simulink model "IslandMode"  (R2022b)
settings: Solver=ode23tb  StartTime=0.0  StopTime=24*3600*365*3  FixedStep=60  RelTol=1e-3
values from neighbouring files (symbols this model uses):
  Fnom = 50    [run_test.m]
  OverChargingProtection = 0    [run_test.m]
  Tsample = 60    [run_test.m]
  Vnom = sqrt(3)*230    [run_test.m]
libraries: simulink x12, ET3036TU_model_library_2021b x7, spsThreePhaseDynamicLoadLib x3, spspowerguiLib x1
settings Model: Creator=nkpanda  LastModifiedBy=jeroen
settings SolverCC: ZeroCrossAlgorithm=Adaptive
settings DebuggingCC: IgnoredZcDiagnostic=none  UnconnectedInputMsg=warning  UnconnectedOutputMsg=warning  UnconnectedLineMsg=warning
settings ModelReferenceCC: EnableRefExpFcnMdlSchedulingChecks=on
settings RTWCC: DLArmComputeVersion=19.05

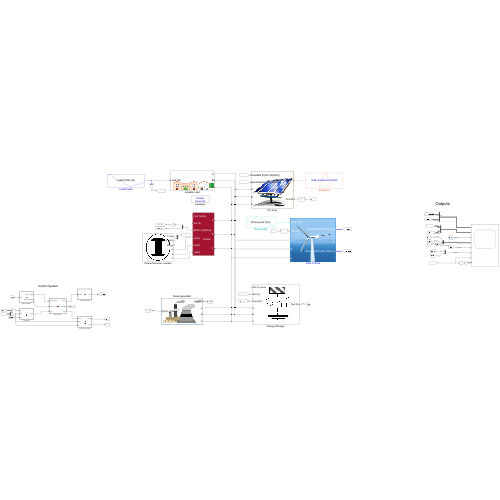
[thumbnail: Simulink's stored preview of the top-level diagram]
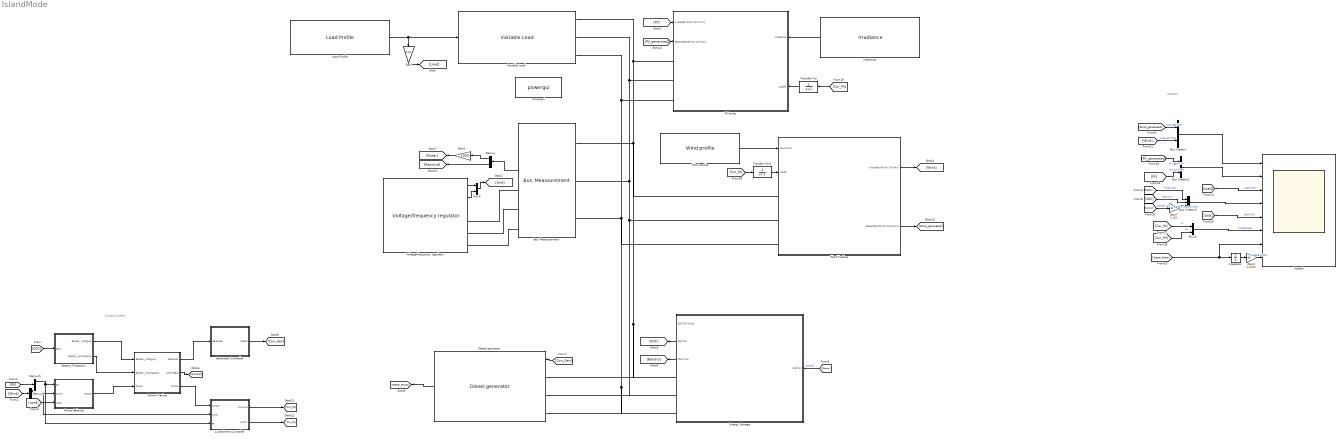
== system IslandMode ==
  note: Control System
  note: Outputs
  Battery Protection : MATLAB Function  TreatAsAtomicUnit=on
  Bus Creator : BusCreator  Inputs=2
  Bus Creator1 : BusCreator  Inputs=2
  Bus Creator2 : BusCreator  Inputs=3
  "Bus Meassurement " : ET3036TU_model_library_2021b/Bus  Meassurement 
  Curtailment Controller : MATLAB Function  TreatAsAtomicUnit=on
  Demux : Demux  Outputs=2
  Demux5 : Demux  Outputs=2
  Demux6 : Demux  Outputs=2
  Diesel generator : ET3036TU_model_library_2021b/Diesel generator  Snom=150  Pfactor=1
  Energy Storage : Subsystem  AncestorBlock=ET3036TU_model_library_2021b/Energy Storage  mask(Grid-connected Energy Storage (PQ Model)){Vn=Vnom, Fn=Fnom, PnomkW=150, kWh_Rated=651.78, Efficiency=100, LimitVec=[90 10], RechargeSOC=70, Precharge=100, autoRecharge=off, Initial_kWh_pc=50, PQvec=[0 0], ovrchargpro=OverChargingProtection}
      mask prompts: Vn "Nominal Line Voltage [Vrms]"; Fn "Nominal Frequency [Hz]"; PnomkW "Rated Power [kW]"; kWh_Rated "Rated Capacity [kWh]"; Efficiency "Overall System Efficiency [%]"; LimitVec "Upper/Lower Charge Limits [%]"; RechargeSOC "SOC to Recharge [%]"; Precharge "Recharge Rate [% of Rated Power]"; autoRecharge "Enable Auto-Recharge"; Initial_kWh_pc "Initial State-of-Charge [0-100%]"; PQvec "Initial Active/Reactive Cmds"; ovrchargpro "Enable over charging/ discharging protection (0: Disable, 1: Enable)"
      mask help:
      | The energy storage block models a generic grid-connected energy storage system (ESS), most commonly a battery system. This is a system-level model that does not contain any power electronics, but is useful for load flow, phasor, and hybrid phasor-EMT simulations. The inputs to this block are the commanded active and reactive power of the ESS.
      |
      | Note: Positive cmd indicates discharging (supply), negative cmd indicates charging (load).
      | Note: The initial active/reactive power commands must be specified for use for Load Flow analysis.
      mask init:
      | % Calculate Initial Conditions
      | Pnom = PnomkW*1e3;
      | P0 = -PQvec(1);  Q0 = -PQvec(2);
      | if abs(P0) > Pnom
      |     P0 = sign(P0)*Pnom;
      | end
      | 
      | % Calculate Q0 given Reactive Power Capability Curve
      | Qlim = sqrt(Pnom^2 - P0^2);
      | if Qlim > abs(Q0)
      |     Q0 = sign(Q0)*Qlim;
      | end
      | 
      | UpChrgLim = LimitVec(1);
      | LowChrgLim = LimitVec(2);
      | if Initial_kWh_pc > UpChrgLim && P0 < 0
      |     P0 = 0; Q0 = 0;
      | elseif Initial_kWh_pc < LowChrgLim && P0 > 0
      |     P0 = 0; Q0 = 0;
      | end
      settings: LibrarySourceBlock=ET3036TU_model_library_2021b/Energy Storage
      mask DialogControl Container7 Prompt: Grid Connection Properties
      mask DialogControl Container11 Prompt: Charge/Discharge Controls
      mask DialogControl Container12 Prompt: Initial Conditions
      mask Display: image('$imagefile'); % Use "Edit Image" on toolstrip to change.
  Gain : Gain  Gain=0.001
  Gain1 : Gain  Gain=1000
  Gain2 : Gain  Gain=1/3600
  Gain7 : Gain  Gain=0.001
  Generator Controller : MATLAB Function  TreatAsAtomicUnit=on
  Integrator : Integrator
  Irradiance : ET3036TU_model_library_2021b/Irradiance
  Load Profile : ET3036TU_model_library_2021b/Load Profile
  Mux4 : Mux  Inputs=2
  Mux5 : Mux  Inputs=2
  "PV array " : Subsystem  AncestorBlock=ET3036TU_model_library_2021b/PV array  mask(PV farm){Efficiency=0.2, Area=822.71, Vnom=Vnom, fnom=Fnom}
      mask prompts: Efficiency "Total efficiency (fraction)"; Area "Area (m2)"; Vnom "Rated Line voltage (Vrms)"; fnom "Rated frequency (Hz):"
      mask help: The product of the efficiency, the area covered by the PV farm and the irradiance in W/m2 will give you the power generated by the PV farm.
      settings: LibrarySourceBlock=ET3036TU_model_library_2021b/PV array
      mask Display:
      | color('white')
      | image(imread('pv.jpg'))
      | 
      | color('black')
      | port_label('RConn',1,'A')
      | port_label('RConn',2,'B')
      | port_label('RConn',3,'C')
      | port_label('output',1,'Available [P(kW) Q(kVAr)]')
      | port_label('output',2,'Generated [P(kW) Q(kVAr)]')
      | 
      | port_label('input',1,'Irradiance (W/m2)')
      | port_label('input',2,'Cut-off')
  Power Balance : MATLAB Function  TreatAsAtomicUnit=on
  Power Tracker : MATLAB Function  TreatAsAtomicUnit=on
  Scope3 : Scope  NumInputPorts=8
  Transfer Fcn : TransferFcn  Denominator=[1 1]
  Transfer Fcn1 : TransferFcn  Denominator=[1 1]
  Variable Load : ET3036TU_model_library_2021b/Variable Load  PF=1  Load0=0
  Voltage/frequency regulator : ET3036TU_model_library_2021b/Voltage//frequency regulator
  "Wind Turbine " : Subsystem  AncestorBlock=ET3036TU_model_library_2021b/Wind Turbine  mask{Unom=15, Umax=25, Umin=3, Pselect=1: Simple Cubic Power, fnom=Fnom, Vnom=Vnom, Pnom=226.56, rp=5, Cp=16/27, rho=1.225, Uvec=1:1:30, Pvec=[0,0,0,0,21359.3750000000,58193.5000000000,104316.125000000,157104.500000000,213935.875000000,272187.500000000,329236.625000000,382460.500000000,429236.375000000,466941.500000000,492953.125000000,500000,500000,500000,500000,500000,500000,500000,500000,500000,500000,0,0,0,0,0], Tp=1, Tq=0.1, ReactP=0}
      mask prompts: Unom "Nominal Wind Speed [m/s]"; Umax "Maximum Operating Wind [m/s]"; Umin "Minimum Operating Wind [m/s]"; Pselect "Wind Turbine Power Model"; fnom "Nominal frequency (Hz):"; Vnom "Nominal phae-to-phase voltage (Vrms)"; Pnom "Nominal Power, [kW]"; rp "Blade Radius, r [m]"; Cp "Performance Coefficient, Cp"; rho "Air Density, rho [kg/m^3]"; Uvec "Wind Vec [m/s]"; Pvec "Power Vec [W]"; Tp "Active Power Dynamics, Tp [s]"; Tq "Reactive Power Dynamics, Tq [s]"; ReactP "Reactive Power Percentage [%]"
      mask help:
      | Simple Wind Turbine that serves as an Active and Reactive Power Source depending on the Wind Power Curve.
      |
      | The Wind Turbine Power Curve can be defined by one of three models:
      | 1: Simple cubic power curve
      | 2: Physical wind turbine parameters
      | 3: Look-up table (from a wind turbine data sheet).
      |
      | Cutoff takes value 1 or 0. 1 denotes manual forced cut-off od wind power generation even though potnetial wind power is available
      | The 'General' and 'Dynamics' tabs apply to all models.
      mask init:
      | A = pi*rp^2;
      | 
      | if Pselect == 1,
      |     Pmax = Pnom*1e3;
      | elseif Pselect == 2,
      |     Pmax = 1/2*rho*Cp*A*Umax^3;
      | else
      |     Pmax = max(Pvec);
      | end
      | Qmax = (ReactP/100)*Pmax;
      settings: LibrarySourceBlock=ET3036TU_model_library_2021b/Wind Turbine
      mask TypeOptions Pselect: 1: Simple Cubic Power | 2: Physical parameters | 3: Look-up Fit
      mask DialogControl Container4 Prompt: General
      mask DialogControl Container16 Prompt: Turbine
      mask DialogControl Container10 Prompt: Electrical
      mask DialogControl Container12 Prompt: 1: Cubic
      mask DialogControl Container9 Prompt: 2: Physical
      mask DialogControl Container7 Prompt: 3: Lookup
      mask DialogControl Container8 Prompt: Dynamics
      mask Display:
      | image(imread('eolienne.bmp'))
      | 
      | color('white')
      | port_label('LConn',1,'A')
      | port_label('LConn',2,'B')
      | port_label('LConn',3,'C')
      | 
      | port_label('output',1,'Available [P(kW) Q(kVAr)]')
      | port_label('output',2,'Generated [P(kW) Q(kVAr)]')
      | port_label('input',1,'Wind (m/s)')
      | port_label('input',2,'Cut-off')
  Wind profile : ET3036TU_model_library_2021b/Wind profile
  powergui : spspowerguiLib/powergui  Priority=1  SimulationMode=Phasor  SampleTime=Tsample  frequency=Fnom  Iterations=50  frequencyindice=50  Pbase=100e6  ErrMax=1e-4  UnitsV=kV  UnitsW=MW  buscounter=0  FunctionMessages=off  echomessages=off  EnableUseOfTLC=off  CurrentSourceSwitches=off  DisableSnubberDevices=off  DisableRonSwitches=off  DisableVfSwitches=off  DisplayEquations=off  AutomaticDiscreteSolvers=off  SolverType=Tustin/Backward Euler (TBE)  Interpol=off  ExternalGateDelay=off  methode=off  Ts=100  x0status=blocks  SPID=on  SwTol=0  HookPort=off  NonlinearTolerance=1e-4  nMaxIteration=100  ContinueOnMaxIteration=off  RestoreLinks=warning  ResistiveCurrentMeasurement=off  Frange=[0:2:500]  Ylog=off  Xlog=on  ShowGrid=off  save=off  variable=ZData  structure=0  ZoomFFT=off  StartTime=0.0  cycles=1  DisplayStyle=1  fundamental=60  FreqAxis=off  MaxFrequency=1000  frequencyindicesteady=1  RmsSteady=1  display=off
  wires:
  Load Profile/1 -> Gain/1, Variable Load/1
  Irradiance/1 -> "PV array "/1(Irradiance)
  Energy Storage/3(Pout (kW)) -> [Battery]
  Energy Storage/2(SOC(%)) -> [SOC]
  Gain/1 -> [Load]
  [Control] -> Energy Storage/1(Pref (W))  "Control"
  Demux/1 -> Gain1/1
  Gain1/1 -> [Power]
  "Bus Meassurement "/3 -> Demux/1
  Demux/2 -> [Reactive]
  [Cur_PV] -> Transfer Fcn/1
  [Cur_W] -> Transfer Fcn1/1
  "PV array "/1(Available [P(kW) Q(kVAr)]) -> [PV]
  "Wind Turbine "/1(Available [P(kW) Q(kVAr)]) -> [Wind]
  Transfer Fcn/1 -> "PV array "/2(cutoff1)
  Transfer Fcn1/1 -> "Wind Turbine "/2(cutoff)
  [Battery] -> Bus Creator2/1  "P_bat (kW)"
  [SOC] -> Bus Creator2/2  "SOC (%)"
  "Wind Turbine "/2(Generated [P(kW) Q(kVAr)]1) -> [Wind_generated]
  "PV array "/2(Generated [P(kW) Q(kVAr)]) -> [PV_generated]
  [Wind_generated] -> Bus Creator/1  "wind_gen(kW)"
  [Wind] -> Bus Creator/2  "wind_act (kW)"
  [PV] -> Bus Creator1/2  "PV_act (kW)"
  [PV_generated] -> Bus Creator1/1  "PV_gen (kW)"
  Bus Creator/1 -> Scope3/1
  Bus Creator1/1 -> Scope3/2
  Bus Creator2/1 -> Scope3/4
  [Control] -> Gain7/1  "Control (W)"
  Gain7/1 -> Bus Creator2/3  "Battery Control (kW)"
  [Cur_W] -> Mux4/1  "W"
  [Cur_PV] -> Mux4/2  "PV"
  Mux4/1 -> Scope3/6  "Curtailment"
  [SOC] -> Battery Protection/1(SOC)
  [Load] -> Power Balance/3(Load)
  Battery Protection/1(Battery_charging) -> Power Tracker/1(Battery_Charging)
  Power Balance/1(Power) -> Power Tracker/3(Power)
  Power Tracker/3(Curtail) -> Curtailment Controller/1(Curtail)
  Power Tracker/1(Generate) -> Generator Controller/1(Generate)
  Curtailment Controller/1(Curwind) -> [Cur_W]
  Curtailment Controller/2(CurPV) -> [Cur_PV]
  [PV] -> Demux5/1
  Demux5/1 -> Curtailment Controller/3(PV), Power Balance/1(Sol)
  [Wind] -> Demux6/1
  Demux6/1 -> Curtailment Controller/2(wind), Power Balance/2(Wind)
  Battery Protection/2(Battery_discharging) -> Power Tracker/2(Battery_discharging)
  [Load] -> Scope3/3  "Load (kW)"
  [Grid] -> Scope3/5  "Grid (kW)"
  Generator Controller/1(Diesel) -> [Con_Gen]
  Diesel generator/1 -> [Diesel_Power]
  [Diesel_Power] -> Scope3/7, Integrator/1
  Wind profile/1 -> "Wind Turbine "/1(Wind (m/s))
  [Con_Gen] -> Diesel generator/1
  Voltage/frequency regulator/1 -> Mux5/1
  Voltage/frequency regulator/2 -> Mux5/2
  Mux5/1 -> [Grid]
  Integrator/1 -> Gain2/1
  Gain2/1 -> Scope3/8  "Diesel (kWh)"
  Power Tracker/2(ControlBat) -> [Control]
  connections:
  "Bus Meassurement "/RConn1 -- Voltage/frequency regulator/RConn1
  "Bus Meassurement "/RConn2 -- Voltage/frequency regulator/RConn2
  "Bus Meassurement "/RConn3 -- Voltage/frequency regulator/RConn3
  "PV array "/RConn2 -- Energy Storage/RConn2 -- Diesel generator/LConn2 -- "Wind Turbine "/LConn2 -- "Bus Meassurement "/LConn2 -- Variable Load/RConn2
  "Bus Meassurement "/LConn1 -- "Wind Turbine "/LConn1 -- Diesel generator/LConn1 -- Energy Storage/RConn1 -- Variable Load/RConn1 -- "PV array "/RConn1
  "PV array "/RConn3 -- "Wind Turbine "/LConn3 -- Diesel generator/LConn3 -- Energy Storage/RConn3 -- "Bus Meassurement "/LConn3 -- Variable Load/RConn3

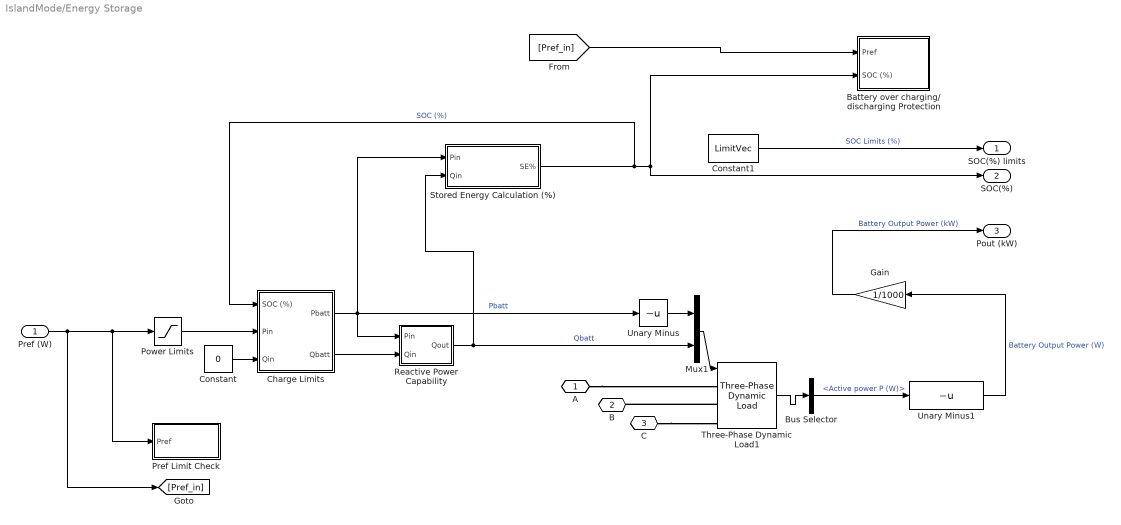
== system IslandMode/Energy Storage ==
  Pref (W) : Inport
  Battery over charging/ discharging Protection : Subsystem
  Bus Selector : BusSelector  OutputSignals=Active power P (W)
  Charge Limits : Subsystem
  Constant : Constant  Value=0
  Constant1 : Constant  Value=LimitVec
  Gain : Gain  Gain=1/1000
  Mux1 : Mux  Inputs=2
  Power Limits : Saturate  UpperLimit=Pnom  LowerLimit=-Pnom
  Pref Limit Check : Subsystem
  Reactive Power Capability : Subsystem
  Stored Energy Calculation (%) : Subsystem
  Three-Phase Dynamic Load1 : spsThreePhaseDynamicLoadLib/Three-Phase Dynamic Load  NominalVoltage=[Vn Fn]  ActiveReactivePowers="[ 0  0]"  PositiveSequence=[Vn 0]  ExternalControl=on  NpNq=[1.3 2]  TimeConstants="[0  0  0  0]"  MinimumVoltage=0.7  Tfilter=1e-4  LoadFlowParameters=[4,0,0,0,0]
  Unary Minus : UnaryMinus
  Unary Minus1 : UnaryMinus
  A : PMIOPort  Side=Right
  B : PMIOPort  Port=2  Side=Right
  C : PMIOPort  Port=3  Side=Right
  SOC(%) limits : Outport  VectorParamsAs1DForOutWhenUnconnected=off
  SOC(%) : Outport  Port=2  VectorParamsAs1DForOutWhenUnconnected=off
  Pout (kW) : Outport  Port=3  VectorParamsAs1DForOutWhenUnconnected=off
  wires:
  Unary Minus/1 -> Mux1/1
  Mux1/1 -> Three-Phase Dynamic Load1/1
  Three-Phase Dynamic Load1/1 -> Bus Selector/1
  Reactive Power Capability/1(Qout) -> Stored Energy Calculation (%)/2(Qin), Mux1/2  "Qbatt"
  Pref (W)/1 -> [Pref_in], Pref Limit Check/1(Pref), Power Limits/1
  Stored Energy Calculation (%)/1(SE%) -> Battery over charging/ discharging Protection/2(SOC (%)), SOC(%)/1, Charge Limits/1(SOC (%))  "SOC (%)"
  Charge Limits/1(Pbatt) -> Stored Energy Calculation (%)/1(Pin), Unary Minus/1, Reactive Power Capability/1(Pin)  "Pbatt"
  Power Limits/1 -> Charge Limits/2(Pin)
  Constant/1 -> Charge Limits/3(Qin)
  Charge Limits/2(Qbatt) -> Reactive Power Capability/2(Qin)
  Bus Selector/1 -> Unary Minus1/1  "<Active power P (W)>"
  Unary Minus1/1 -> Gain/1  "Battery Output Power (W)"
  Gain/1 -> Pout (kW)/1  "Battery Output Power (kW)"
  [Pref_in] -> Battery over charging/ discharging Protection/1(Pref)
  Constant1/1 -> SOC(%) limits/1  "SOC Limits (%)"
  connections:
  Three-Phase Dynamic Load1/LConn2 -- B/RConn1
  C/RConn1 -- Three-Phase Dynamic Load1/LConn3
  A/RConn1 -- Three-Phase Dynamic Load1/LConn1

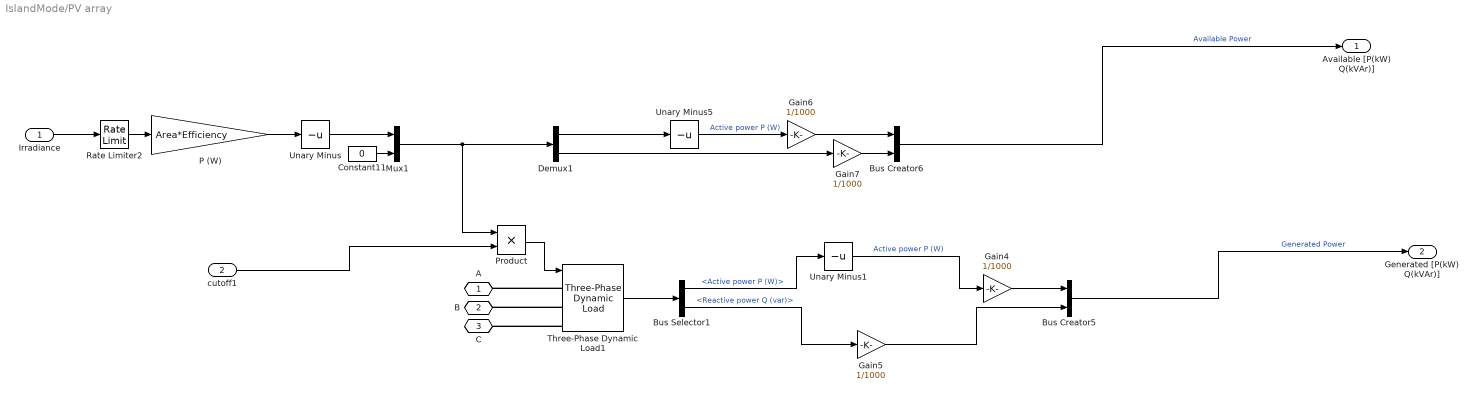
== system IslandMode/PV array  ==
  Irradiance : Inport
  cutoff1 : Inport  Port=2
  Bus Creator5 : BusCreator  Inputs=2
  Bus Creator6 : BusCreator  Inputs=2
  Bus Selector1 : BusSelector  OutputSignals=Active power P (W),Reactive power Q (var)
  Constant11 : Constant  Value=0
  Demux1 : Demux  Outputs=2
  Gain{4..7} (4 alike) : Gain  Gain=1/1000
  Mux1 : Mux  Inputs=2
  P (W) : Gain  Gain=Area*Efficiency
  Product : Product
  Rate Limiter2 : RateLimiter  RisingSlewLimit=1e4  FallingSlewLimit=-1e4  SampleTimeMode=inherited
  Three-Phase Dynamic Load1 : spsThreePhaseDynamicLoadLib/Three-Phase Dynamic Load  NominalVoltage=[Vnom fnom]  ActiveReactivePowers="[ 0  0]"  PositiveSequence=[Vnom 0]  ExternalControl=on  NpNq=[1.3 2]  TimeConstants="[0  0  0  0]"  MinimumVoltage=0.7  Tfilter=1e-4  LoadFlowParameters=[4,0,0,0,0]
  Unary Minus : UnaryMinus
  Unary Minus1 : UnaryMinus
  Unary Minus5 : UnaryMinus
  A : PMIOPort  Side=Right
  B : PMIOPort  Port=2  Side=Right
  C : PMIOPort  Port=3  Side=Right
  Available [P(kW) Q(kVAr)] : Outport  VectorParamsAs1DForOutWhenUnconnected=off
  Generated [P(kW) Q(kVAr)] : Outport  Port=2  VectorParamsAs1DForOutWhenUnconnected=off
  wires:
  Bus Creator5/1 -> Generated [P(kW) Q(kVAr)]/1  "Generated Power"
  Rate Limiter2/1 -> P (W)/1
  Constant11/1 -> Mux1/2
  Unary Minus/1 -> Mux1/1
  P (W)/1 -> Unary Minus/1
  Irradiance/1 -> Rate Limiter2/1
  Bus Selector1/1 -> Unary Minus1/1  "<Active power P (W)>"
  Unary Minus1/1 -> Gain4/1  "Active power P (W)"
  Three-Phase Dynamic Load1/1 -> Bus Selector1/1
  Bus Selector1/2 -> Gain5/1  "<Reactive power Q (var)>"
  Gain4/1 -> Bus Creator5/1
  Gain5/1 -> Bus Creator5/2
  Demux1/1 -> Unary Minus5/1
  Gain6/1 -> Bus Creator6/1
  Demux1/2 -> Gain7/1
  Unary Minus5/1 -> Gain6/1  "Active power P (W)"
  Gain7/1 -> Bus Creator6/2
  Bus Creator6/1 -> Available [P(kW) Q(kVAr)]/1  "Available Power"
  Product/1 -> Three-Phase Dynamic Load1/1
  Mux1/1 -> Product/1, Demux1/1
  cutoff1/1 -> Product/2
  connections:
  Three-Phase Dynamic Load1/LConn2 -- B/RConn1
  Three-Phase Dynamic Load1/LConn1 -- A/RConn1
  Three-Phase Dynamic Load1/LConn3 -- C/RConn1

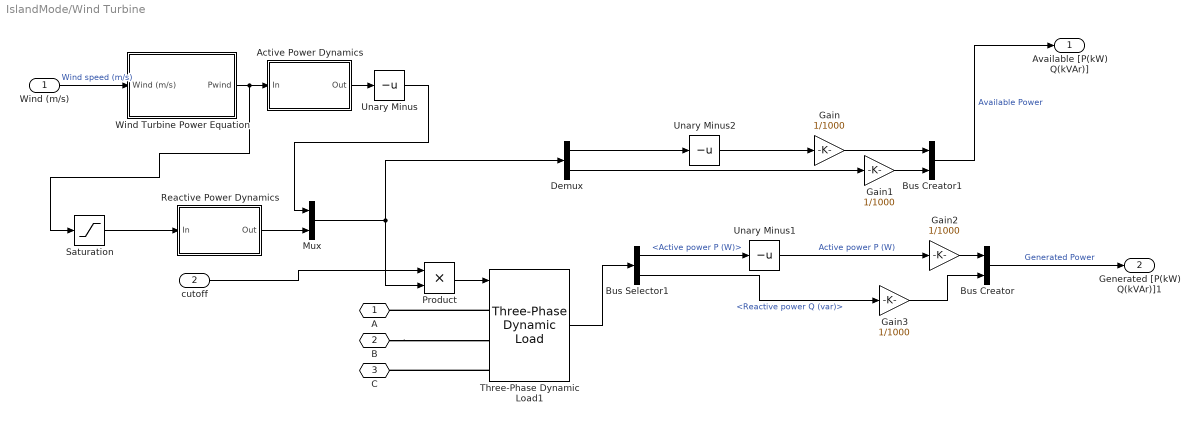
== system IslandMode/Wind Turbine  ==
  Wind (m/s) : Inport
  cutoff : Inport  Port=2
  Active Power Dynamics : Subsystem  VariantControl=T6NotZero
      mask Display: disp('1 / (1 + s T_P)','texmode','on');
  Bus Creator : BusCreator  Inputs=2
  Bus Creator1 : BusCreator  Inputs=2
  Bus Selector1 : BusSelector  OutputSignals=Active power P (W),Reactive power Q (var)
  Demux : Demux  Outputs=2
  Gain{,1..3} (4 alike) : Gain  Gain=1/1000
  Mux : Mux  Inputs=2
  Product : Product
  Reactive Power Dynamics : Subsystem  VariantControl=T6NotZero
      mask Display: disp('1 / (1 + s T_Q)','texmode','on');
  Saturation : Saturate  UpperLimit=Qmax  LowerLimit=-Qmax
  Three-Phase Dynamic Load1 : spsThreePhaseDynamicLoadLib/Three-Phase Dynamic Load  NominalVoltage=[Vnom fnom]  ActiveReactivePowers="[ 0  0]"  PositiveSequence=[Vnom 0]  ExternalControl=on  NpNq=[1.3 2]  TimeConstants="[0  0  0  0]"  MinimumVoltage=0.7  Tfilter=1e-4  LoadFlowParameters=[4,0,0,0,0]
  Unary Minus : UnaryMinus
  Unary Minus1 : UnaryMinus
  Unary Minus2 : UnaryMinus
  Wind Turbine Power Equation : Subsystem
  A : PMIOPort  Side=Left
  B : PMIOPort  Port=2  Side=Left
  C : PMIOPort  Port=3  Side=Left
  Available [P(kW) Q(kVAr)] : Outport  VectorParamsAs1DForOutWhenUnconnected=off
  Generated [P(kW) Q(kVAr)]1 : Outport  Port=2  VectorParamsAs1DForOutWhenUnconnected=off
  wires:
  Bus Selector1/2 -> Gain3/1  "<Reactive power Q (var)>"
  Unary Minus1/1 -> Gain2/1  "Active power P (W)"
  Bus Selector1/1 -> Unary Minus1/1  "<Active power P (W)>"
  Three-Phase Dynamic Load1/1 -> Bus Selector1/1
  Unary Minus/1 -> Mux/1
  Active Power Dynamics/1(Out) -> Unary Minus/1
  Wind Turbine Power Equation/1(Pwind) -> Saturation/1, Active Power Dynamics/1(In)
  Reactive Power Dynamics/1(Out) -> Mux/2
  Saturation/1 -> Reactive Power Dynamics/1(In)
  Wind (m/s)/1 -> Wind Turbine Power Equation/1(Wind (m/s))  "Wind speed (m/s)"
  Mux/1 -> Demux/1, Product/2
  Product/1 -> Three-Phase Dynamic Load1/1
  cutoff/1 -> Product/1
  Demux/1 -> Unary Minus2/1
  Demux/2 -> Gain1/1
  Unary Minus2/1 -> Gain/1
  Gain/1 -> Bus Creator1/1
  Gain1/1 -> Bus Creator1/2
  Gain2/1 -> Bus Creator/1
  Gain3/1 -> Bus Creator/2
  Bus Creator1/1 -> Available [P(kW) Q(kVAr)]/1  "Available Power"
  Bus Creator/1 -> Generated [P(kW) Q(kVAr)]1/1  "Generated Power"
  connections:
  B/RConn1 -- Three-Phase Dynamic Load1/LConn2
  Three-Phase Dynamic Load1/LConn3 -- C/RConn1
  Three-Phase Dynamic Load1/LConn1 -- A/RConn1

== system IslandMode/Energy Storage/Battery over charging// discharging Protection ==
  Pref : Inport
  SOC (%) : Inport  Port=2
  Over Charging Protection : Subsystem
  Under Charging Protection : Subsystem
  wires:
  SOC (%)/1 -> Under Charging Protection/1(SOC (%)), Over Charging Protection/1(SOC (%))
  Pref/1 -> Under Charging Protection/2(Pref), Over Charging Protection/2(Pref)

== system IslandMode/Energy Storage/Charge Limits ==
  SOC (%) : Inport
  Pin : Inport  Port=2
  Qin : Inport  Port=3
  Overcharge Check : Subsystem
  Undercharge Check : Subsystem
  Pbatt : Outport  VectorParamsAs1DForOutWhenUnconnected=off
  Qbatt : Outport  Port=2  VectorParamsAs1DForOutWhenUnconnected=off
  wires:
  Overcharge Check/2(Qout) -> Undercharge Check/3(Qin)
  Undercharge Check/1(Pout) -> Pbatt/1  "Pbatt"
  Qin/1 -> Overcharge Check/3(Qin)
  Overcharge Check/1(Pout) -> Undercharge Check/2(Pin)
  Pin/1 -> Overcharge Check/2(Pin)
  Undercharge Check/2(Qout) -> Qbatt/1
  SOC (%)/1 -> Undercharge Check/1(SOC (%)), Overcharge Check/1(SOC (%))

== system IslandMode/Energy Storage/Pref Limit Check ==
  Pref : Inport
  Abs1 : Abs  SaturateOnIntegerOverflow=off
  Constant1 : Constant  Value=PnomkW
  Gain : Gain  Gain=1000
  Simulation Stop : MATLAB Function  TreatAsAtomicUnit=on
  Subtract : Sum  Inputs=+-
  wires:
  Subtract/1 -> Simulation Stop/1(u)
  Abs1/1 -> Subtract/2
  Constant1/1 -> Gain/1
  Pref/1 -> Abs1/1
  Gain/1 -> Subtract/1

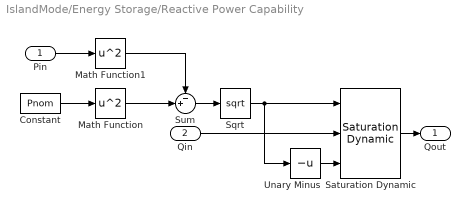
== system IslandMode/Energy Storage/Reactive Power Capability ==
  Pin : Inport
  Qin : Inport  Port=2
  Constant : Constant  Value=Pnom
  Math Function : Math  Operator=square  SignedPower=on
  Math Function1 : Math  Operator=square  SignedPower=on
  Saturation Dynamic : simulink/Discontinuities/Saturation Dynamic  OutMin=[]  OutMax=[]  OutDataTypeStr=Inherit: Same as second input  OutDataType=fixdt(1, 16)  OutScaling=2^-10  DoSatur=off
  Sqrt : Sqrt
  Sum : Sum  Inputs=-+|
  Unary Minus : UnaryMinus
  Qout : Outport  VectorParamsAs1DForOutWhenUnconnected=off
  wires:
  Qin/1 -> Saturation Dynamic/2
  Pin/1 -> Math Function1/1
  Saturation Dynamic/1 -> Qout/1
  Unary Minus/1 -> Saturation Dynamic/3
  Sum/1 -> Sqrt/1
  Constant/1 -> Math Function/1
  Math Function/1 -> Sum/2
  Math Function1/1 -> Sum/1
  Sqrt/1 -> Unary Minus/1, Saturation Dynamic/1

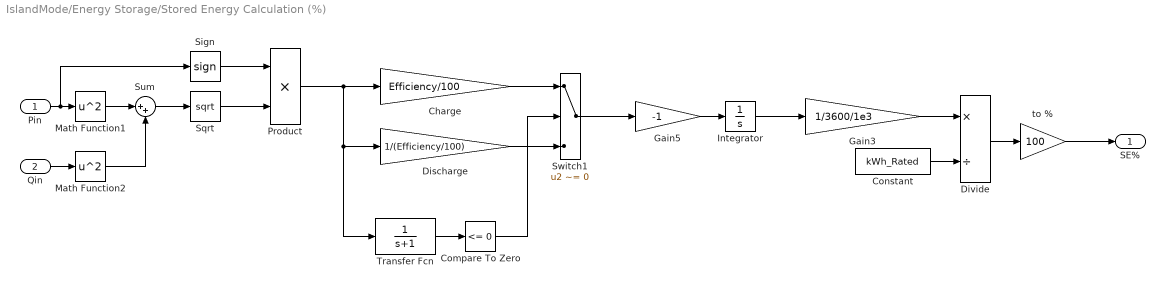
== system IslandMode/Energy Storage/Stored Energy Calculation (%) ==
  Pin : Inport
  Qin : Inport  Port=2
  Charge : Gain  Gain=Efficiency/100
  Compare To Zero : simulink/Logic and Bit Operations/Compare To Zero  relop=<=  OutDataTypeStr=boolean
  Constant : Constant  Value=kWh_Rated
  Discharge : Gain  Gain=1/(Efficiency/100)
  Divide : Product  Inputs=*/
  Gain3 : Gain  Gain=1/3600/1e3
  Gain5 : Gain  Gain=-1
  Integrator : Integrator  InitialCondition=(Initial_kWh_pc/100)*kWh_Rated*3600*1e3
  Math Function1 : Math  Operator=square  SignedPower=on
  Math Function2 : Math  Operator=square  SignedPower=on
  Product : Product
  Sign : Signum
  Sqrt : Sqrt
  Sum : Sum  Inputs=|++
  Switch1 : Switch  Criteria=u2 ~= 0  SaturateOnIntegerOverflow=off  InputSameDT=off
  Transfer Fcn : TransferFcn  Denominator=[1 1]
  to % : Gain  Gain=100
  SE% : Outport  VectorParamsAs1DForOutWhenUnconnected=off
  wires:
  Integrator/1 -> Gain3/1
  Compare To Zero/1 -> Switch1/2
  Divide/1 -> to %/1
  Charge/1 -> Switch1/1
  Constant/1 -> Divide/2
  Gain3/1 -> Divide/1
  Switch1/1 -> Gain5/1
  Transfer Fcn/1 -> Compare To Zero/1
  to %/1 -> SE%/1
  Gain5/1 -> Integrator/1
  Discharge/1 -> Switch1/3
  Product/1 -> Charge/1, Discharge/1, Transfer Fcn/1
  Pin/1 -> Sign/1, Math Function1/1
  Qin/1 -> Math Function2/1
  Math Function1/1 -> Sum/1
  Math Function2/1 -> Sum/2
  Sum/1 -> Sqrt/1
  Sqrt/1 -> Product/2
  Sign/1 -> Product/1

== system IslandMode/Wind Turbine /Active Power Dynamics ==
  In : Inport
  1/Tp : Gain  Gain=1/Tp
  Integrator : Integrator
  Sum : Sum  Inputs=|+-
  Out : Outport  VectorParamsAs1DForOutWhenUnconnected=off
  wires:
  Integrator/1 -> Out/1, Sum/2
  In/1 -> Sum/1
  1/Tp/1 -> Integrator/1
  Sum/1 -> 1/Tp/1

== system IslandMode/Wind Turbine /Reactive Power Dynamics ==
  In : Inport
  1/Tq : Gain  Gain=1/Tq
  Integrator : Integrator
  Sum : Sum  Inputs=|+-
  Out : Outport  VectorParamsAs1DForOutWhenUnconnected=off
  wires:
  Sum/1 -> 1/Tq/1
  1/Tq/1 -> Integrator/1
  In/1 -> Sum/1
  Integrator/1 -> Sum/2, Out/1

== system IslandMode/Wind Turbine /Wind Turbine Power Equation ==
  Wind (m/s) : Inport
  Constant : Constant  Value=Pselect
  Cubic Power with Cutoff : Subsystem
  Manufacturer Fit : Lookup_n-D  NumberOfTableDimensions=1  BreakpointsForDimension1=Uvec  Table=Pvec  ExtrapMethod=Clip  InternalRulePriority=Speed  RndMeth=Simplest
  Multiport Switch : MultiPortSwitch  SaturateOnIntegerOverflow=off  InputSameDT=off
  Saturation : Saturate  UpperLimit=inf  LowerLimit=0  ZeroCross=off
      settings: AttributesFormatString=|
      | %<UpperLimit>
      | %<LowerLimit>
  Wind Turbine Properties : Subsystem
  Pwind : Outport  VectorParamsAs1DForOutWhenUnconnected=off
  wires:
  Manufacturer Fit/1 -> Multiport Switch/4
  Saturation/1 -> Manufacturer Fit/1, Wind Turbine Properties/1(Wind (m/s)), Cubic Power with Cutoff/1(Wind (m/s))
  Constant/1 -> Multiport Switch/1
  Multiport Switch/1 -> Pwind/1
  Wind (m/s)/1 -> Saturation/1
  Wind Turbine Properties/1(Pwind) -> Multiport Switch/3
  Cubic Power with Cutoff/1(Pwind) -> Multiport Switch/2

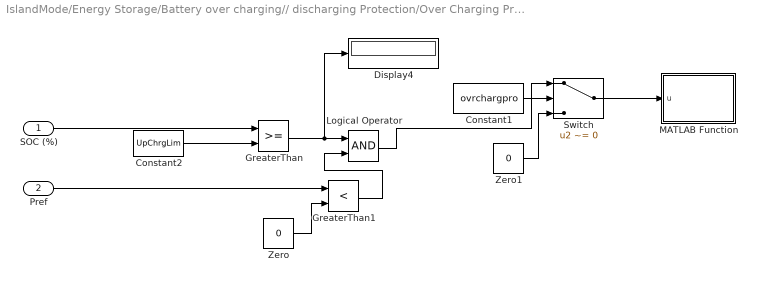
== system IslandMode/Energy Storage/Battery over charging// discharging Protection/Over Charging Protection ==
  SOC (%) : Inport
  Pref : Inport  Port=2
  Constant1 : Constant  Value=ovrchargpro
  Constant2 : Constant  Value=UpChrgLim
  Display4 : Display
  GreaterThan : RelationalOperator  OutDataTypeStr=boolean  RndMeth=Simplest  InputSameDT=off
  GreaterThan1 : RelationalOperator  Operator=<  OutDataTypeStr=boolean  RndMeth=Simplest  InputSameDT=off
  Logical Operator : Logic  AllPortsSameDT=off  OutDataTypeStr=boolean
  MATLAB Function : MATLAB Function  TreatAsAtomicUnit=on
  Switch : Switch  Criteria=u2 ~= 0  SaturateOnIntegerOverflow=off  InputSameDT=off
  Zero : Constant  Value=0  OutDataTypeStr=Inherit: Inherit via back propagation
  Zero1 : Constant  Value=0  OutDataTypeStr=Inherit: Inherit via back propagation
  wires:
  Pref/1 -> GreaterThan1/1
  GreaterThan/1 -> Display4/1, Logical Operator/1
  Logical Operator/1 -> Switch/1
  Constant2/1 -> GreaterThan/2
  GreaterThan1/1 -> Logical Operator/2
  SOC (%)/1 -> GreaterThan/1
  Zero/1 -> GreaterThan1/2
  Switch/1 -> MATLAB Function/1(u)
  Constant1/1 -> Switch/2
  Zero1/1 -> Switch/3

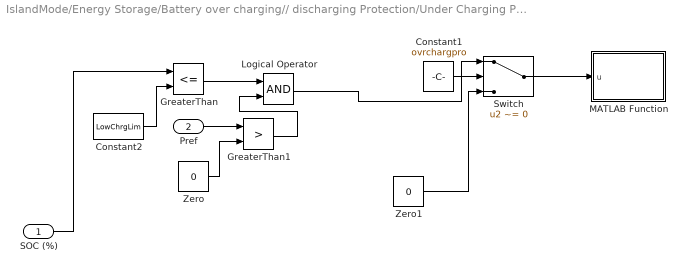
== system IslandMode/Energy Storage/Battery over charging// discharging Protection/Under Charging Protection ==
  SOC (%) : Inport
  Pref : Inport  Port=2
  Constant1 : Constant  Value=ovrchargpro
  Constant2 : Constant  Value=LowChrgLim
  GreaterThan : RelationalOperator  Operator=<=  OutDataTypeStr=boolean  RndMeth=Simplest  InputSameDT=off
  GreaterThan1 : RelationalOperator  Operator=>  OutDataTypeStr=boolean  RndMeth=Simplest  InputSameDT=off
  Logical Operator : Logic  AllPortsSameDT=off  OutDataTypeStr=boolean
  MATLAB Function : MATLAB Function  TreatAsAtomicUnit=on
  Switch : Switch  Criteria=u2 ~= 0  SaturateOnIntegerOverflow=off  InputSameDT=off
  Zero : Constant  Value=0  OutDataTypeStr=Inherit: Inherit via back propagation
  Zero1 : Constant  Value=0  OutDataTypeStr=Inherit: Inherit via back propagation
  wires:
  SOC (%)/1 -> GreaterThan/1
  Zero/1 -> GreaterThan1/2
  GreaterThan1/1 -> Logical Operator/2
  Constant2/1 -> GreaterThan/2
  GreaterThan/1 -> Logical Operator/1
  Pref/1 -> GreaterThan1/1
  Switch/1 -> MATLAB Function/1(u)
  Constant1/1 -> Switch/2
  Zero1/1 -> Switch/3
  Logical Operator/1 -> Switch/1

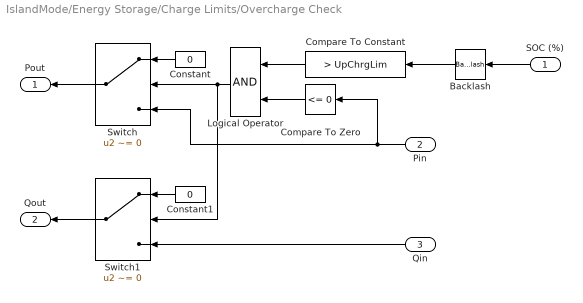
== system IslandMode/Energy Storage/Charge Limits/Overcharge Check ==
  SOC (%) : Inport
  Pin : Inport  Port=2
  Qin : Inport  Port=3
  Backlash : Backlash  BacklashWidth=1e-3  InitialOutput=Initial_kWh_pc  ZeroCross=off
  Compare To Constant : simulink/Logic and Bit Operations/Compare To Constant  relop=>  const=UpChrgLim  OutDataTypeStr=boolean
  Compare To Zero : simulink/Logic and Bit Operations/Compare To Zero  relop=<=  OutDataTypeStr=boolean
  Constant : Constant  Value=0
  Constant1 : Constant  Value=0
  Logical Operator : Logic  AllPortsSameDT=off  OutDataTypeStr=boolean
  Switch : Switch  Criteria=u2 ~= 0  SaturateOnIntegerOverflow=off  InputSameDT=off
  Switch1 : Switch  Criteria=u2 ~= 0  SaturateOnIntegerOverflow=off  InputSameDT=off
  Pout : Outport  VectorParamsAs1DForOutWhenUnconnected=off
  Qout : Outport  Port=2  VectorParamsAs1DForOutWhenUnconnected=off
  wires:
  Compare To Constant/1 -> Logical Operator/1
  Logical Operator/1 -> Switch1/2, Switch/2
  Constant/1 -> Switch/1
  SOC (%)/1 -> Backlash/1
  Pin/1 -> Compare To Zero/1, Switch/3
  Switch/1 -> Pout/1
  Compare To Zero/1 -> Logical Operator/2
  Qin/1 -> Switch1/3
  Constant1/1 -> Switch1/1
  Switch1/1 -> Qout/1
  Backlash/1 -> Compare To Constant/1

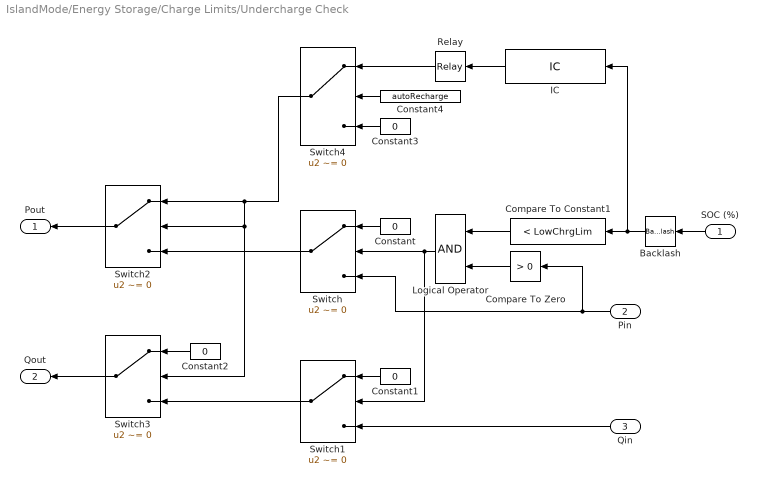
== system IslandMode/Energy Storage/Charge Limits/Undercharge Check ==
  SOC (%) : Inport
  Pin : Inport  Port=2
  Qin : Inport  Port=3
  Backlash : Backlash  BacklashWidth=1e-3  InitialOutput=Initial_kWh_pc  ZeroCross=off
  Compare To Constant1 : simulink/Logic and Bit Operations/Compare To Constant  relop=<  const=LowChrgLim  OutDataTypeStr=boolean
  Compare To Zero : simulink/Logic and Bit Operations/Compare To Zero  relop=>  OutDataTypeStr=boolean
  Constant{,1..3} (4 alike) : Constant  Value=0
  Constant4 : Constant  Value=autoRecharge
  IC : InitialCondition  Value=RechargeSOC
  Logical Operator : Logic  AllPortsSameDT=off  OutDataTypeStr=boolean
  Relay : Relay  OnSwitchValue=RechargeSOC  OffSwitchValue=LowChrgLim  OnOutputValue=0  OffOutputValue=-Precharge/100*Pnom
  Switch{,1..4} (5 alike) : Switch  Criteria=u2 ~= 0  SaturateOnIntegerOverflow=off  InputSameDT=off
  Pout : Outport  VectorParamsAs1DForOutWhenUnconnected=off
  Qout : Outport  Port=2  VectorParamsAs1DForOutWhenUnconnected=off
  wires:
  Compare To Zero/1 -> Logical Operator/2
  Pin/1 -> Switch/3, Compare To Zero/1
  SOC (%)/1 -> Backlash/1
  Constant/1 -> Switch/1
  Logical Operator/1 -> Switch/2, Switch1/2
  Compare To Constant1/1 -> Logical Operator/1
  Constant1/1 -> Switch1/1
  Qin/1 -> Switch1/3
  Backlash/1 -> IC/1, Compare To Constant1/1
  Switch4/1 -> Switch2/1, Switch2/2, Switch3/2
  IC/1 -> Relay/1
  Switch/1 -> Switch2/3
  Switch2/1 -> Pout/1
  Switch3/1 -> Qout/1
  Switch1/1 -> Switch3/3
  Constant2/1 -> Switch3/1
  Relay/1 -> Switch4/1
  Constant3/1 -> Switch4/3
  Constant4/1 -> Switch4/2

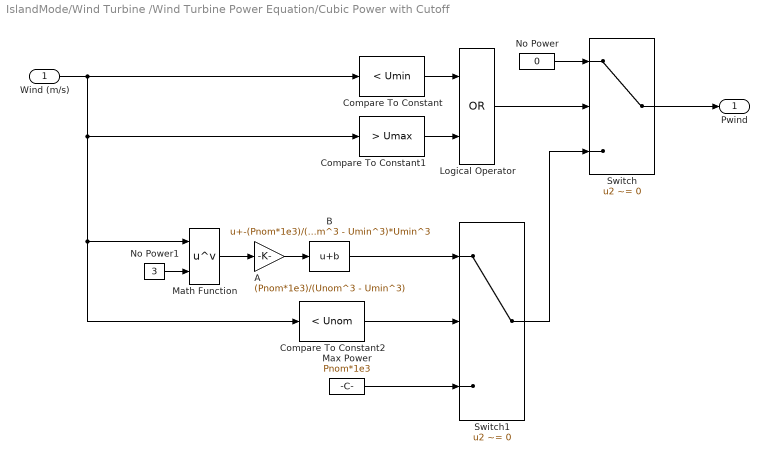
== system IslandMode/Wind Turbine /Wind Turbine Power Equation/Cubic Power with Cutoff ==
  Wind (m/s) : Inport
  A : Gain  Gain=(Pnom*1e3)/(Unom^3 - Umin^3)
  B : Bias  Bias=-(Pnom*1e3)/(Unom^3 - Umin^3)*Umin^3  SaturateOnIntegerOverflow=off
  Compare To Constant : simulink/Logic and Bit Operations/Compare To Constant  relop=<  const=Umin  OutDataTypeStr=boolean
  Compare To Constant1 : simulink/Logic and Bit Operations/Compare To Constant  relop=>  const=Umax  OutDataTypeStr=boolean
  Compare To Constant2 : simulink/Logic and Bit Operations/Compare To Constant  relop=<  const=Unom  OutDataTypeStr=boolean
  Logical Operator : Logic  Operator=OR  AllPortsSameDT=off  OutDataTypeStr=boolean
  Math Function : Math  Operator=pow  SignedPower=on
  Max Power : Constant  Value=Pnom*1e3
  No Power : Constant  Value=0
  No Power1 : Constant  Value=3
  Switch : Switch  Criteria=u2 ~= 0  ZeroCross=off  SaturateOnIntegerOverflow=off  InputSameDT=off
  Switch1 : Switch  Criteria=u2 ~= 0  ZeroCross=off  SaturateOnIntegerOverflow=off  InputSameDT=off
  Pwind : Outport  VectorParamsAs1DForOutWhenUnconnected=off
  wires:
  Compare To Constant/1 -> Logical Operator/1
  Switch/1 -> Pwind/1
  Logical Operator/1 -> Switch/2
  A/1 -> B/1
  Wind (m/s)/1 -> Compare To Constant2/1, Math Function/1, Compare To Constant1/1, Compare To Constant/1
  Max Power/1 -> Switch1/3
  Switch1/1 -> Switch/3
  No Power/1 -> Switch/1
  No Power1/1 -> Math Function/2
  Math Function/1 -> A/1
  Compare To Constant1/1 -> Logical Operator/2
  Compare To Constant2/1 -> Switch1/2
  B/1 -> Switch1/1

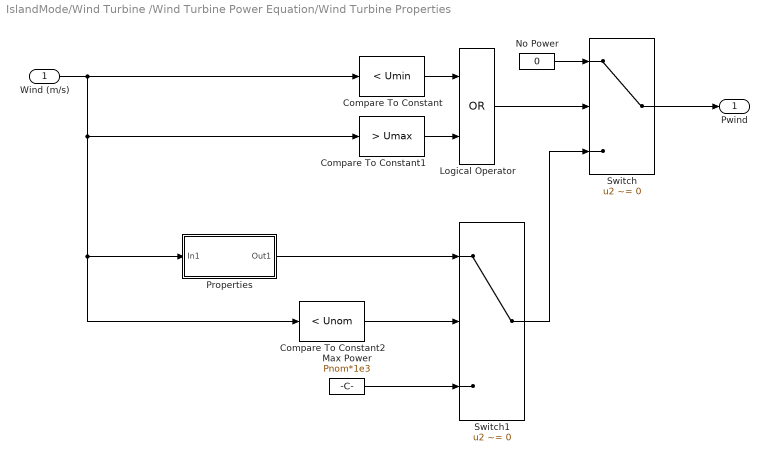
== system IslandMode/Wind Turbine /Wind Turbine Power Equation/Wind Turbine Properties ==
  Wind (m/s) : Inport
  Compare To Constant : simulink/Logic and Bit Operations/Compare To Constant  relop=<  const=Umin  OutDataTypeStr=boolean
  Compare To Constant1 : simulink/Logic and Bit Operations/Compare To Constant  relop=>  const=Umax  OutDataTypeStr=boolean
  Compare To Constant2 : simulink/Logic and Bit Operations/Compare To Constant  relop=<  const=Unom  OutDataTypeStr=boolean
  Logical Operator : Logic  Operator=OR  AllPortsSameDT=off  OutDataTypeStr=boolean
  Max Power : Constant  Value=Pnom*1e3
  No Power : Constant  Value=0
  Properties : Subsystem
  Switch : Switch  Criteria=u2 ~= 0  ZeroCross=off  SaturateOnIntegerOverflow=off  InputSameDT=off
  Switch1 : Switch  Criteria=u2 ~= 0  ZeroCross=off  SaturateOnIntegerOverflow=off  InputSameDT=off
  Pwind : Outport  VectorParamsAs1DForOutWhenUnconnected=off
  wires:
  Properties/1(Out1) -> Switch1/1
  Compare To Constant2/1 -> Switch1/2
  Compare To Constant1/1 -> Logical Operator/2
  No Power/1 -> Switch/1
  Switch1/1 -> Switch/3
  Max Power/1 -> Switch1/3
  Wind (m/s)/1 -> Compare To Constant/1, Compare To Constant1/1, Properties/1(In1), Compare To Constant2/1
  Logical Operator/1 -> Switch/2
  Switch/1 -> Pwind/1
  Compare To Constant/1 -> Logical Operator/1

== system IslandMode/Wind Turbine /Wind Turbine Power Equation/Wind Turbine Properties/Properties ==
  In1 : Inport
  Air Density : Gain  Gain=rho
  Blade Swept Area (m^2) : Gain  Gain=A
  Gain : Gain  Gain=1/2
  Power Coefficient : Constant  Value=Cp
  "Product " : Product  SaturateOnIntegerOverflow=on  OutDataTypeStr=Inherit: Same as first input
  wind_speed^3 : Fcn  Expr=u(1)^3
  Out1 : Outport  VectorParamsAs1DForOutWhenUnconnected=off
  wires:
  Blade Swept Area (m^2)/1 -> "Product "/1
  wind_speed^3/1 -> Air Density/1
  Power Coefficient/1 -> "Product "/2
  In1/1 -> wind_speed^3/1
  Air Density/1 -> Gain/1
  "Product "/1 -> Out1/1
  Gain/1 -> Blade Swept Area (m^2)/1

== matlab function IslandMode/Energy Storage/Battery over charging// discharging Protection/Over Charging Protection/MATLAB Function ==
  data: u input
function fcn(u)
    if u == 1
        error('Battery is fully charged (Max SOC% reached), hence cannot charge more. Increase SOC% or Check Pref signal')
    end

== matlab function IslandMode/Energy Storage/Battery over charging// discharging Protection/Under Charging Protection/MATLAB Function ==
  data: u input
function fcn(u)
    if u == 1
        error('Battery is discharged fully (Min SOC% reached), hence cannot discharge more. Decrease SOC% or Check Pref signal')
    end

== matlab function IslandMode/Energy Storage/Pref Limit Check/Simulation Stop ==
  data: u input
function  fcn(u)
if u<0
    error('Power reference to the battery exceeds the battery''s nominal power')
end

== matlab function IslandMode/Power Balance ==
  data: Sol input; Power output; Wind input; Load input
%Calculate how much power is short or access
function Power  = fcn(Sol, Wind, Load)
Power = Sol*1000 + Wind*1000 - Load*1000;

== matlab function IslandMode/Power Tracker ==
  data: Battery_Charging input; Battery_discharging input; Power input; Generate output; ControlBat output; Curtail output
function [Generate,ControlBat, Curtail]  = fcn(Battery_Charging, Battery_discharging, Power)
%Determines how much power is too short or too much
if Power > 0 %Too much power available
    Curtail = Power - Battery_Charging*1000;
    if Curtail <= 0
        ControlBat = -(Battery_Charging*1000 +Curtail);
       else
        ControlBat = -Battery_Charging*1000;
    end
    Generate = 0;
else %Too little power available
    Curtail = 0;
    Generate = Power + Battery_discharging*1000;
    if Generate >= 0
        ControlBat = (Battery_discharging*1000 -Generate);
    else
        ControlBat = Battery_discharging*1000;
    end
end

== matlab function IslandMode/Battery Protection ==
  data: SOC input; Battery_charging output; Battery_discharging output
function [Battery_charging, Battery_discharging]   = fcn(SOC)
fill = SOC/100;
%Calculate how much power the battery can maximumly charge or discharge.
Prated = 100; %kW
bounds = [0.1,0.90]; %Maximum charge and drainage of the battery
Capacity = 350; %kWh
Capacity_upper = Capacity*bounds(2); %kWh
Capacity_lower = Capacity*bounds(1); %kWh

if fill*Capacity+Prated >= Capacity_upper
    Battery_charging = Capacity_upper - fill*Capacity;
    Battery_discharging = Prated;
elseif fill*Capacity-Prated <= Capacity_lower
    Battery_discharging = fill*Capacity - Capacity_lower;
    Battery_charging = Prated;
else
    Battery_charging = Prated;
    Battery_discharging = Prated;
end

== matlab function IslandMode/Curtailment Controller ==
  data: Curtail input; Curwind output; CurPV output; wind input; PV input
function [Curwind, CurPV]  = fcn(Curtail,wind,PV)
%Determines how much each source needs to be curtailed
Win = wind*1000;
PVin = PV*1000;
R_pv = PVin/(PVin+Win);
R_w = 1-R_pv;
if Curtail <= 0
    CurPV = 1;
    Curwind = 1;
else
    if PVin <= 0.0001
        Curwind = (Win - R_w*Curtail)/Win;
        CurPV =1;
    elseif Win <= 0.0001
        CurPV = (PVin- R_pv*Curtail)/PVin;
        Curwind = 1;
    else
        Curwind = (Win - R_w*Curtail)/Win;
        CurPV = (PVin- R_pv*Curtail)/PVin;
    end
end

== matlab function IslandMode/Generator Controller ==
  data: Generate input; Diesel output
function Diesel    = fcn(Generate)
%Determines how much power is too short or too much
if Generate >= 0
    Diesel = 0;
else
    Diesel = -Generate;
end
